simulink model "fangzhen20200803"  (Simulink 9.0)
settings: Solver=ode4  StartTime=0.0  StopTime=500  FixedStep=0.05  RelTol=1e-3
InitFcn:
  | data
values from neighbouring files (symbols this model uses):
  A = [1    0     0 ... (first row only)    [cx.m]    (also in data.m = [Wex^2-W^2   Wex*Wey    Wex*Wez; data1.m = [Wex^2-W^2   Wex*Wey    Wex*Wez)
  a = F/m0    (= 0.2)    [data.m]    (also in data1.m = 0.02)
  a0 = 2*a*k/(4*a+k)    (= 0.08)    [data.m]    (also in data1.m = 0.00363636363636)
  AWcc = [1 1 1]*0.15/3600/3*pi/180    [data.m]    (also in data1.m)
  B = [   0    -2*Wez    2*Wey ... (first row only)    [data.m]    (also in data1.m)
  b = 0.00001*(a+a0)/(2*a*a0)    (= 8.75e-05)    [data.m]    (also in data1.m = 0.01625)
  c20 = -0.113    [data.m]    (also in data1.m)
  c22 = 0.0396    [data.m]    (also in data1.m)
  CWw = [1,1,1,1]*6e-5    [data.m]    (also in data1.m)
  d = 0.01    [data.m]    (also in data1.m = 0.1)
  DWN = [sin(bata)*cos(alpha)  sin(bata)*sin(alpha)  -sin(bata)*cos(alpha)  -sin(bata)*sin(alpha) ... (first row only)    [data.m]    (also in data1.m)
  f = f+2*pi    [E2C.m]    (also in data.m = -0.02; data1.m = 0.02)
  Gl = [-cos(xit0)*sin(fai0)   sin(xit0)*sin(fai0)    cos(fai0) ... (first row only)    [data.m]    (also in data1.m)
  HBd0 = IBd*We0    [data.m]    (also in data1.m)
  Hwmax = JW.*Wwmax    [data.m]    (also in data1.m)
  HWw0 = [0.01 0.01 0.01 0.01]    [data.m]    (also in data1.m)
  InvIBd = inv(IBd)    [data.m]    (also in data1.m)
  invJW = 1 ./JW    [data.m]    (also in data1.m)
  Isp = 300*9.8    (= 2940)    [data.m]    (also in data1.m)
  IW = [1,1,1,1]*1.e-6    [data.m]    (also in data1.m)
  JW = [1,1,1,1]*0.0017362    [data.m]    (also in data1.m)
  Kd = [19.2895;16.6643;22.1166]    [data.m]    (also in data1.m)
  Ki = [0.0503;0.0503;0.0503]    [data.m]    (also in data1.m)
  Kp = [7.0313;6.0484;8.0898]    [data.m]    (also in data1.m)
  m0 = 200    [data.m]    (also in data1.m)
  Mu = 4.794e3    (= 4794)    [data.m]    (also in data1.m)
  MWN = DWN'*inv(DWN*DWN')    [data.m]    (also in data1.m)
  Noise_gc = [1 -1 1]*6/3600*pi/180    [data.m]    (also in data1.m)
  Noise_gn = ([1 1 1]*0.0025/3.*pi/180).^2    [data.m]    (also in data1.m)
  Noise_rwn = ([1 1 1].*1e-10).^2    [data.m]    (also in data1.m)
  Qb0 = [QQQ(4);QQQ(1:3)]    [data.m]    (also in data1.m)
  r0 = [100;-200;1000]    [data.m]    (also in data1.m = [200;300;1000])
  R0 = Tl*[0;0;R0l]    [data.m]    (also in data1.m)
  re = 1750    [data.m]    (also in data1.m)
  rg0 = [3;-104;950]    [data.m]    (also in data1.m = [203;292;998])
  Rtb = [0;0;0]    [data.m]    (also in data1.m = [-30;50;0])
  T = 200    [data.m]    (also in data1.m = 1200)
  TA = [0 0 0]'    [data.m]    (also in data1.m)
  TB = [500 0 0]'    [data.m]    (also in data1.m)
  TC = [500 500 0]'    [data.m]    (also in data1.m)
  Tcmax = [1,1,1,1].*0.02    [data.m]    (also in data1.m)
  TWf0 = [1,1,1,1]*3e-4    [data.m]    (also in data1.m)
  v0 = [-0.1;0.1;-0.3]    [data.m]    (also in data1.m = [0.1;0.1;-1.0])
  vg0 = [0;-0.1;-0.4]    [data.m]    (also in data1.m = [0;-0.1;-0.7])
  Wcc = [1 1 1]*0.2    [data.m]    (also in data1.m)
  We = Tl*Gl'*[0;0;W]    [data.m]    (also in data1.m)
  Wgmax = 10*[1,1,1]'*pi/180    [data.m]    (also in data1.m)
undefined symbols (not defined in the file or in its folder): DiscIntNeverNeededParam, HB0, magnitude
libraries: sharedtransform x4, aerolibobsolete x4, sharedutil x1
(part 1 of 2)
settings Model: SuppressorTable=22 serialization::archive 11 0 6 0 0 0 0 0  Creator=Administrator  LastModifiedBy=chenshiming
settings DataIOCC: LimitDataPoints=on  SignalLoggingSaveFormat=ModelDataLogs  SignalLoggingName=sigsOut
settings OptimizationCC: BlockReduction=off  DefaultParameterBehavior=Inlined  BufferReuse=off  ExpressionDepthLimit=2147483647
settings DebuggingCC: SaveWithParameterizedLinksMsg=none  SignalResolutionControl=TryResolveAllWithWarning  MultiTaskDSMMsg=warning  MultiTaskCondExecSysMsg=none  StateNameClashWarn=warning  StrictBusMsg=None
settings HardwareCC: TargetBitPerLong=64  TargetBitPerPointer=64  TargetBitPerSizeT=64  TargetBitPerPtrDiffT=64  TargetLongLongMode=on  TargetIntDivRoundTo=Zero  TargetEndianess=LittleEndian  TargetWordSize=64  TargetHWDeviceType=MATLAB Host  ProdEqTarget=off
settings GRTTargetCC: GeneratePreprocessorConditionals=Disable all  CombineOutputUpdateFcns=off  GRTInterface=on

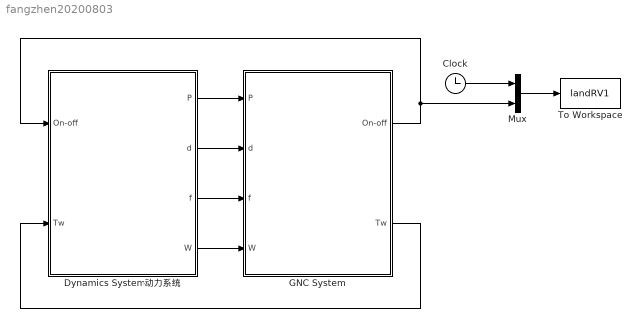
== system fangzhen20200803 ==
  Clock : Clock
  Dynamics System动力系统 : Subsystem
  GNC System : Subsystem
  Mux : Mux  Inputs=2
  To Workspace : ToWorkspace  VariableName=landRV1  SampleTime=-1
  wires:
  Dynamics System动力系统/1(P) -> GNC System/1(P)
  Dynamics System动力系统/2(d) -> GNC System/2(d)
  Dynamics System动力系统/3(f) -> GNC System/3(f)
  Dynamics System动力系统/4(W) -> GNC System/4(W)
  GNC System/1(On-off) -> Dynamics System动力系统/1(On-off), Mux/2
  GNC System/2(Tw) -> Dynamics System动力系统/2(Tw)
  Clock/1 -> Mux/1
  Mux/1 -> To Workspace/1

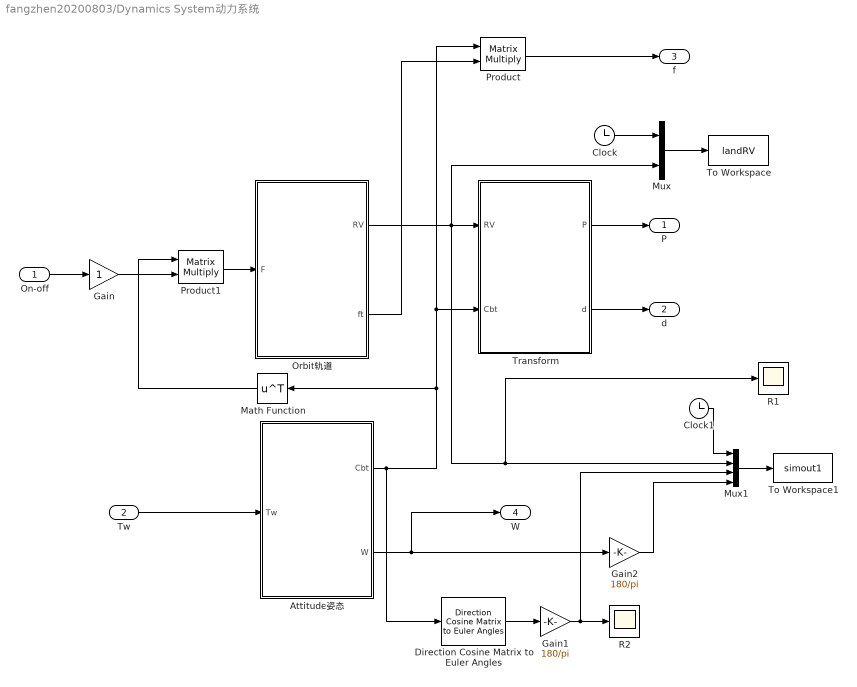
== system fangzhen20200803/Dynamics System动力系统 ==
  On-off : Inport
  Tw : Inport  Port=2
  Attitude姿态 : Subsystem
  Clock : Clock
  Clock1 : Clock
  Direction Cosine Matrix to Euler Angles : aerolibobsolete/Direction Cosine Matrix to Euler Angles
      settings: SourceProductName=Aerospace Blockset  SourceProductBaseCode=AE
  Gain : Gain  SaturateOnIntegerOverflow=on  OutDataTypeStr=Inherit: Same as input  ParamDataTypeStr=Inherit: Same as input
  Gain1 : Gain  Gain=180/pi  SaturateOnIntegerOverflow=on  OutDataTypeStr=Inherit: Same as input  ParamDataTypeStr=Inherit: Same as input
  Gain2 : Gain  Gain=180/pi  SaturateOnIntegerOverflow=on  OutDataTypeStr=Inherit: Same as input  ParamDataTypeStr=Inherit: Same as input
  Math Function : Math  Operator=transpose  SaturateOnIntegerOverflow=on
  Mux : Mux  Inputs=2
  Mux1 : Mux
  Orbit轨道 : Subsystem
  Product : Product  Multiplication=Matrix(*)  SaturateOnIntegerOverflow=on  OutDataTypeStr=Inherit: Same as first input
  Product1 : Product  Multiplication=Matrix(*)  SaturateOnIntegerOverflow=on  OutDataTypeStr=Inherit: Same as first input
  R1 : Scope
  R2 : Scope
  To Workspace : ToWorkspace  VariableName=landRV  SampleTime=-1
  To Workspace1 : ToWorkspace  VariableName=simout1  SampleTime=-1
  Transform : Subsystem
  P : Outport
  d : Outport  Port=2
  f : Outport  Port=3
  W : Outport  Port=4
  wires:
  Tw/1 -> Attitude姿态/1(Tw)
  Attitude姿态/1(Cbt) -> Product/1, Transform/2(Cbt), Math Function/1, Direction Cosine Matrix to Euler Angles/1
  Orbit轨道/2(ft) -> Product/2
  Product/1 -> f/1
  Attitude姿态/2(W) -> W/1, Gain2/1
  Orbit轨道/1(RV) -> R1/1, Mux1/2, Mux/2, Transform/1(RV)
  Transform/2(d) -> d/1
  Transform/1(P) -> P/1
  On-off/1 -> Gain/1
  Product1/1 -> Orbit轨道/1(F)
  Gain/1 -> Product1/2
  Math Function/1 -> Product1/1
  Direction Cosine Matrix to Euler Angles/1 -> Gain1/1
  Gain1/1 -> R2/1, Mux1/3
  Clock/1 -> Mux/1
  Mux/1 -> To Workspace/1
  Clock1/1 -> Mux1/1
  Mux1/1 -> To Workspace1/1
  Gain2/1 -> Mux1/4

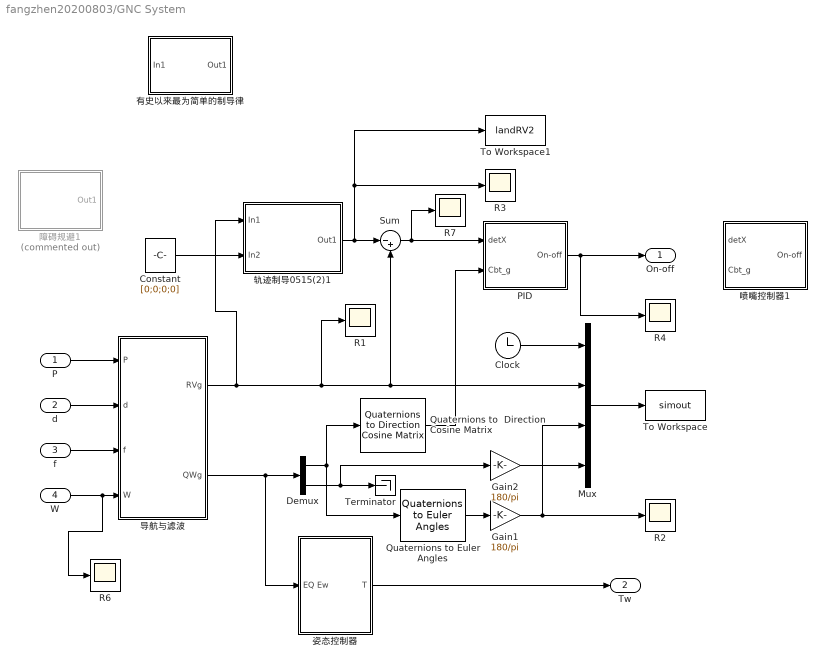
== system fangzhen20200803/GNC System ==
  P : Inport
  d : Inport  Port=2
  f : Inport  Port=3
  W : Inport  Port=4
  Clock : Clock
  Constant : Constant  Value=[0;0;0;0]  VectorParams1D=off
  Demux : Demux  Outputs=[4 3]
  Gain1 : Gain  Gain=180/pi  SaturateOnIntegerOverflow=on  OutDataTypeStr=Inherit: Same as input  ParamDataTypeStr=Inherit: Same as input
  Gain2 : Gain  Gain=180/pi  SaturateOnIntegerOverflow=on  OutDataTypeStr=Inherit: Same as input  ParamDataTypeStr=Inherit: Same as input
  Mux : Mux
  "PID " : Subsystem
  Quaternions to  Direction Cosine Matrix : sharedtransform/Quaternions to  Direction Cosine Matrix
      settings: SourceProductName=Aerospace Blockset  SourceProductBaseCode=AE
  Quaternions to Euler Angles : aerolibobsolete/Quaternions to Euler Angles
      settings: SourceProductName=Aerospace Blockset  SourceProductBaseCode=AE
  R{1..4,6..7} (6 alike) : Scope
  Sum : Sum  Inputs=|-+  SaturateOnIntegerOverflow=on
  Terminator : Terminator
  To Workspace : ToWorkspace  VariableName=simout  SampleTime=-1
  To Workspace1 : ToWorkspace  VariableName=landRV2  SampleTime=-1
  喷嘴控制器1 : Subsystem
  姿态控制器 : Subsystem
      mask help:
      | 输入:
      | 偏差四元数与偏差角速度(本体系下)
      | 输出:
      | 控制电压
      mask Display: disp('姿态控制器')
  导航与滤波 : Subsystem
  "有史以来最为简单的制导律 " : Subsystem
  轨迹制导0515(2)1 : Subsystem
      mask Display: disp('轨迹制导')
  障碍规避1 : Subsystem  Commented=on
      mask Display: disp('障碍规避')
  On-off : Outport
  Tw : Outport  Port=2
  wires:
  P/1 -> 导航与滤波/1(P)
  d/1 -> 导航与滤波/2(d)
  f/1 -> 导航与滤波/3(f)
  W/1 -> R6/1, 导航与滤波/4(W)
  导航与滤波/2(QWg) -> Demux/1, 姿态控制器/1(EQ Ew)
  姿态控制器/1(T) -> Tw/1
  导航与滤波/1(RVg) -> 轨迹制导0515(2)1/1(In1), R1/1, Sum/2, Mux/2
  Demux/2 -> Terminator/1, Gain2/1
  Demux/1 -> Quaternions to  Direction Cosine Matrix/1, Quaternions to Euler Angles/1
  Quaternions to  Direction Cosine Matrix/1 -> "PID "/2(Cbt_g)
  "PID "/1(On-off) -> On-off/1, R4/1
  Quaternions to Euler Angles/1 -> Gain1/1
  Gain1/1 -> R2/1, Mux/3
  Clock/1 -> Mux/1
  Mux/1 -> To Workspace/1
  Gain2/1 -> Mux/4
  Sum/1 -> R7/1, "PID "/1(detX)
  轨迹制导0515(2)1/1(Out1) -> To Workspace1/1, R3/1, Sum/1
  Constant/1 -> 轨迹制导0515(2)1/2(In2)

== system fangzhen20200803/Dynamics System动力系统/Attitude姿态 ==
  Tw : Inport
  Constant : Constant  Value=We
  Product : Product  Multiplication=Matrix(*)  SaturateOnIntegerOverflow=on  OutDataTypeStr=Inherit: Same as first input
  Quaternions to  Direction Cosine Matrix : sharedtransform/Quaternions to  Direction Cosine Matrix
      settings: SourceProductName=Aerospace Blockset  SourceProductBaseCode=AE
  Sum1 : Sum  Inputs=+-  SaturateOnIntegerOverflow=on
  反作用飞轮 : Subsystem
      mask help:
      | 输入:
      | 1、控制信号(力矩形式)
      | 2、星体绝对角速度(本体系下)
      | 输出:
      | 反作用力矩(本体系下)
      mask Display: disp('反作用飞轮')
  姿态动力学模型 : Subsystem
      mask help:
      | 输入:
      | 作用力矩(本体系下)
      | 输出:
      | 绝对角速度(本体系下)
      mask Display: disp('姿态动力学模型')
  星体运动学 : Subsystem  mask(Kinemitics Mask){}
      mask help:
      | 输入:
      | 本体系相对特征点系的角速度(本体系下)
      | 输出:
      | 本体系相对特征点系的姿态四元数
      mask Display: disp('姿态运动学\n(四元数)')
  Cbt : Outport
  W : Outport  Port=2
  wires:
  Tw/1 -> 反作用飞轮/1(Uwheel)
  Quaternions to  Direction Cosine Matrix/1 -> Product/1, Cbt/1
  Constant/1 -> Product/2
  Product/1 -> Sum1/2
  姿态动力学模型/1(Wb) -> Sum1/1, 反作用飞轮/2(Wb), W/1
  Sum1/1 -> 星体运动学/1(In2)
  星体运动学/1(Out2) -> Quaternions to  Direction Cosine Matrix/1
  反作用飞轮/1(TW) -> 姿态动力学模型/1(Torque)

== system fangzhen20200803/Dynamics System动力系统/Orbit轨道 ==
  F : Inport
  轨道动力学模型 : Subsystem
      mask help:
      | 输入:
      | 喷嘴产生的推力(特征点坐标系)
      | 输出:
      | 1、探测器的位置与速度(特征点坐标系)
      | 2、比力(特征点坐标系)
      mask Display: disp('轨道动力学模型')
  RV : Outport
  ft : Outport  Port=2
  wires:
  F/1 -> 轨道动力学模型/1(F)
  轨道动力学模型/1(X) -> RV/1
  轨道动力学模型/2(bl) -> ft/1

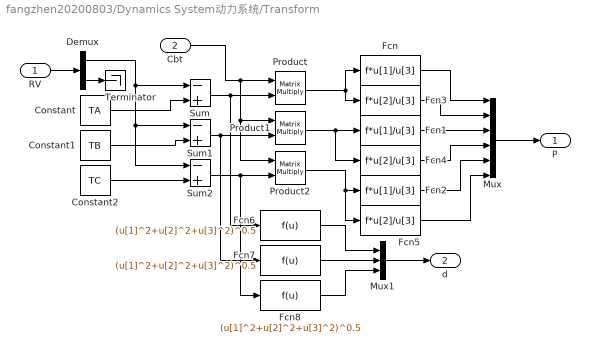
== system fangzhen20200803/Dynamics System动力系统/Transform ==
  RV : Inport
  Cbt : Inport  Port=2
  Constant : Constant  Value=TA
  Constant1 : Constant  Value=TB
  Constant2 : Constant  Value=TC
  Demux : Demux  Outputs=[3 3]
  Fcn : Fcn  Expr=f*u[1]/u[3]
  Fcn1 : Fcn  Expr=f*u[1]/u[3]
  Fcn2 : Fcn  Expr=f*u[1]/u[3]
  Fcn3 : Fcn  Expr=f*u[2]/u[3]
  Fcn4 : Fcn  Expr=f*u[2]/u[3]
  Fcn5 : Fcn  Expr=f*u[2]/u[3]
  Fcn6 : Fcn  Expr=(u[1]^2+u[2]^2+u[3]^2)^0.5
  Fcn7 : Fcn  Expr=(u[1]^2+u[2]^2+u[3]^2)^0.5
  Fcn8 : Fcn  Expr=(u[1]^2+u[2]^2+u[3]^2)^0.5
  Mux : Mux  Inputs=6
  Mux1 : Mux  Inputs=3
  Product : Product  Multiplication=Matrix(*)  SaturateOnIntegerOverflow=on  OutDataTypeStr=Inherit: Same as first input
  Product1 : Product  Multiplication=Matrix(*)  SaturateOnIntegerOverflow=on  OutDataTypeStr=Inherit: Same as first input
  Product2 : Product  Multiplication=Matrix(*)  SaturateOnIntegerOverflow=on  OutDataTypeStr=Inherit: Same as first input
  Sum : Sum  Inputs=-+  SaturateOnIntegerOverflow=on
  Sum1 : Sum  Inputs=-+  SaturateOnIntegerOverflow=on
  Sum2 : Sum  Inputs=-+  SaturateOnIntegerOverflow=on
  Terminator : Terminator
  P : Outport
  d : Outport  Port=2
  wires:
  RV/1 -> Demux/1
  Demux/2 -> Terminator/1
  Demux/1 -> Sum/1, Sum2/1, Sum1/1
  Constant/1 -> Sum/2
  Constant1/1 -> Sum1/2
  Constant2/1 -> Sum2/2
  Cbt/1 -> Product/1, Product2/1, Product1/1
  Sum/1 -> Product/2, Fcn6/1
  Sum1/1 -> Product1/2, Fcn7/1
  Sum2/1 -> Product2/2, Fcn8/1
  Product/1 -> Fcn/1, Fcn3/1
  Product1/1 -> Fcn1/1, Fcn4/1
  Product2/1 -> Fcn2/1, Fcn5/1
  Mux/1 -> P/1
  Fcn7/1 -> Mux1/2
  Fcn8/1 -> Mux1/3
  Fcn6/1 -> Mux1/1
  Mux1/1 -> d/1
  Fcn/1 -> Mux/1
  Fcn3/1 -> Mux/2
  Fcn1/1 -> Mux/3
  Fcn4/1 -> Mux/4
  Fcn2/1 -> Mux/5
  Fcn5/1 -> Mux/6

== system fangzhen20200803/GNC System/PID  ==
  detX : Inport
  Cbt_g : Inport  Port=2
  Delay : Delay  DelayLength=1  InitialCondition=0  SampleTime=0.05
  Demux : Demux  Outputs=[3 3]
  KD : Gain  Gain=0.01
  KD1 : Gain  Gain=-1
  KP : Gain  Gain=0.0002
  Ki : Gain  Gain=0.03  SaturateOnIntegerOverflow=on  OutDataTypeStr=Inherit: Same as input  ParamDataTypeStr=Inherit: Same as input
  Product : Product  Multiplication=Matrix(*)  SaturateOnIntegerOverflow=on  OutDataTypeStr=Inherit: Same as first input
  Product2 : Product  Multiplication=Matrix(*)  SaturateOnIntegerOverflow=on  OutDataTypeStr=Inherit: Same as first input
  Saturation : Saturate  UpperLimit=[0.01,;0.01; 0.01]  LowerLimit=[-0.01; -0.01; -0.01]
  Scope : Scope
  Scope1 : Scope
  Sum1 : Sum  Inputs=|+|+|  SaturateOnIntegerOverflow=on  InputSameDT=on  OutDataTypeStr=Inherit: Same as first input
  Sum2 : Sum  Inputs=|+|+|+|  SaturateOnIntegerOverflow=on  InputSameDT=on  OutDataTypeStr=Inherit: Same as first input
  Zero-Order Hold : ZeroOrderHold  SampleTime=0.05
  On-off : Outport
  wires:
  detX/1 -> Scope/1, Zero-Order Hold/1
  Demux/1 -> Product/2
  Cbt_g/1 -> Product/1, Product2/1
  Demux/2 -> Product2/2
  Sum2/1 -> On-off/1
  Zero-Order Hold/1 -> KD1/1, Scope1/1
  Product2/1 -> KD/1
  Product/1 -> Sum1/2, KP/1, Delay/1
  Sum1/1 -> Ki/1
  Ki/1 -> Saturation/1
  KD/1 -> Sum2/3
  KP/1 -> Sum2/2
  Delay/1 -> Sum1/1
  Saturation/1 -> Sum2/1
  KD1/1 -> Demux/1

== system fangzhen20200803/GNC System/喷嘴控制器1 ==
  detX : Inport
  Cbt_g : Inport  Port=2
  Clock : Clock
  Constant : Constant  Value=T
  Constant3 : Constant  Value=[(2*a*a0/(a+a0)*b)^0.5;(2*a*a0/(a+a0)*b)^0.5;(2*a*a0/(a+a0)*b)^0.5]
  Demux : Demux  Outputs=[3 3]
  Gain : Gain  Gain=-1  SaturateOnIntegerOverflow=on  OutDataTypeStr=Inherit: Same as input  ParamDataTypeStr=Inherit: Same as input
  Product : Product  Multiplication=Matrix(*)  SaturateOnIntegerOverflow=on  OutDataTypeStr=Inherit: Same as first input
  Product2 : Product  Multiplication=Matrix(*)  SaturateOnIntegerOverflow=on  OutDataTypeStr=Inherit: Same as first input
  Product3 : Product  SaturateOnIntegerOverflow=on  OutDataTypeStr=Inherit: Same as first input
  Relational Operator : RelationalOperator  Operator=<=  RndMeth=Nearest
  Relational Operator3 : RelationalOperator  RndMeth=Nearest
  Relational Operator4 : RelationalOperator  RndMeth=Nearest
  Scope : Scope
  Scope1 : Scope
  Sum1 : Sum  SaturateOnIntegerOverflow=on
  Zero-Order Hold : ZeroOrderHold  SampleTime=0.05
  detR+ : Subsystem
  detR- : Subsystem
  On-off : Outport
  wires:
  Gain/1 -> Relational Operator3/2
  Relational Operator3/1 -> detR-/3(change)
  Relational Operator4/1 -> detR+/3(change)
  detR-/1(-T) -> Sum1/1
  detR+/1(+T) -> Sum1/2
  Constant3/1 -> Gain/1, Relational Operator4/2
  Sum1/1 -> Product3/1
  detX/1 -> Scope/1, Zero-Order Hold/1
  Demux/1 -> Product/2
  Cbt_g/1 -> Product/1, Product2/1
  Product/1 -> detR-/1(detR), detR+/1(detR)
  Demux/2 -> Product2/2
  Product2/1 -> Relational Operator4/1, Relational Operator3/1, detR-/2(detV), detR+/2(detV)
  Clock/1 -> Relational Operator/1
  Constant/1 -> Relational Operator/2
  Relational Operator/1 -> Product3/2
  Product3/1 -> On-off/1
  Zero-Order Hold/1 -> Scope1/1, Demux/1

== system fangzhen20200803/GNC System/姿态控制器 ==
  note: 期望力矩
  note: 飞轮分配力矩
  note: 四元数矢量
  EQ Ew : Inport
  Constant1 : Constant  Value=[0 0 0]
  Demux : Demux  Outputs=[1 3]
  Demux1 : Demux  Outputs=[4 3]
  Discrete-Time Integrator : DiscreteIntegrator  IntegratorMethod=Integration: Backward Euler  InitialConditionSource=external  SampleTime=0.2  ICPrevOutput=DiscIntNeverNeededParam  ICPrevScaledInput=DiscIntNeverNeededParam
  Gain : Gain  Gain=[-1 -1 -1]  SaturateOnIntegerOverflow=on  OutDataTypeStr=Inherit: Same as input  ParamDataTypeStr=Inherit: Same as input
  Kd : Gain  Gain=Kd  SaturateOnIntegerOverflow=on  OutDataTypeStr=Inherit: Same as input  ParamDataTypeStr=Inherit: Same as input
  Ki : Gain  Gain=Ki  SaturateOnIntegerOverflow=on  OutDataTypeStr=Inherit: Same as input  ParamDataTypeStr=Inherit: Same as input
  Kp : Gain  Gain=Kp  SaturateOnIntegerOverflow=on  OutDataTypeStr=Inherit: Same as input  ParamDataTypeStr=Inherit: Same as input
  MWN : Gain  Gain=MWN  Multiplication=Matrix(K*u)  SaturateOnIntegerOverflow=on  OutDataTypeStr=Inherit: Same as input  ParamDataTypeStr=Inherit: Same as input
  Product5 : Product  OutDataTypeStr=double  SaturateOnIntegerOverflow=on  InputSameDT=on
  R1 : Scope
  Saturation : Saturate  UpperLimit=[0.01, 0.01, 0.01]  LowerLimit=[-0.01, -0.01, -0.01]
  Sign : Signum
  Sum : Sum  Inputs=+-  SaturateOnIntegerOverflow=on  InputSameDT=on  OutDataTypeStr=Inherit: Same as first input
  Sum1 : Sum  Inputs=+-  SaturateOnIntegerOverflow=on  InputSameDT=on  OutDataTypeStr=Inherit: Same as first input
  Sum2 : Sum  Inputs=|+|+|+|  SaturateOnIntegerOverflow=on  InputSameDT=on  OutDataTypeStr=Inherit: Same as first input
  Terminator : Terminator
  T : Outport
  wires:
  Sum/1 -> Discrete-Time Integrator/1, Kp/1
  Sum1/1 -> Kd/1
  Discrete-Time Integrator/1 -> Ki/1
  Ki/1 -> Saturation/1
  Kp/1 -> Sum2/2
  Kd/1 -> Sum2/3
  Demux/2 -> Product5/2
  Demux/1 -> Sign/1
  Product5/1 -> Sum/2
  Constant1/1 -> Discrete-Time Integrator/2, Sum1/1, Sum/1
  Sum2/1 -> R1/1, Gain/1
  Demux1/2 -> Sum1/2
  Demux1/1 -> Demux/1
  EQ Ew/1 -> Demux1/1
  Sign/1 -> Product5/1
  Saturation/1 -> Terminator/1, Sum2/1
  MWN/1 -> T/1
  Gain/1 -> MWN/1

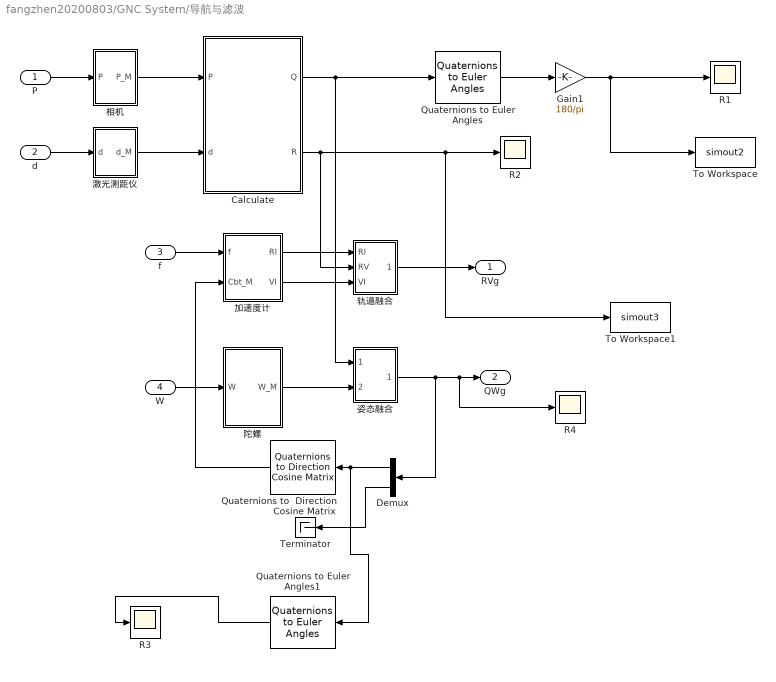
== system fangzhen20200803/GNC System/导航与滤波 ==
  P : Inport
  d : Inport  Port=2
  f : Inport  Port=3
  W : Inport  Port=4
  Calculate : Subsystem
  Demux : Demux  Outputs=[4 3]
  Gain1 : Gain  Gain=180/pi  SaturateOnIntegerOverflow=on  OutDataTypeStr=Inherit: Same as input  ParamDataTypeStr=Inherit: Same as input
  Quaternions to  Direction Cosine Matrix : sharedtransform/Quaternions to  Direction Cosine Matrix
      settings: SourceProductName=Aerospace Blockset  SourceProductBaseCode=AE
  Quaternions to Euler Angles : aerolibobsolete/Quaternions to Euler Angles
      settings: SourceProductName=Aerospace Blockset  SourceProductBaseCode=AE
  Quaternions to Euler Angles1 : aerolibobsolete/Quaternions to Euler Angles
      settings: SourceProductName=Aerospace Blockset  SourceProductBaseCode=AE
  R{1..4} (4 alike) : Scope
  Terminator : Terminator
  To Workspace : ToWorkspace  VariableName=simout2  SampleTime=-1
  To Workspace1 : ToWorkspace  VariableName=simout3  SampleTime=-1
  加速度计 : Subsystem
  姿态融合 : Subsystem
  激光测距仪 : Subsystem
  相机 : Subsystem
  轨道融合 : Subsystem
  陀螺 : Subsystem
  RVg : Outport
  QWg : Outport  Port=2
  wires:
  f/1 -> 加速度计/1(f)
  W/1 -> 陀螺/1(W)
  加速度计/1(RI) -> 轨道融合/1(RI)
  加速度计/2(VI) -> 轨道融合/3(VI)
  Calculate/2(R) -> 轨道融合/2(RV), To Workspace1/1, R2/1
  Calculate/1(Q) -> 姿态融合/1(Q-M), Quaternions to Euler Angles/1
  陀螺/1(W_M) -> 姿态融合/2(w-M)
  轨道融合/1(RVg) -> RVg/1
  姿态融合/1(QWg) -> R4/1, QWg/1, Demux/1
  Demux/1 -> Quaternions to Euler Angles1/1, Quaternions to  Direction Cosine Matrix/1
  Quaternions to  Direction Cosine Matrix/1 -> 加速度计/2(Cbt_M)
  Demux/2 -> Terminator/1
  Quaternions to Euler Angles/1 -> Gain1/1
  Gain1/1 -> R1/1, To Workspace/1
  d/1 -> 激光测距仪/1(d)
  P/1 -> 相机/1(P)
  相机/1(P_M) -> Calculate/1(P)
  激光测距仪/1(d_M) -> Calculate/2(d)
  Quaternions to Euler Angles1/1 -> R3/1

== system fangzhen20200803/GNC System/有史以来最为简单的制导律  ==
  In1 : Inport
  Clock1 : Clock
  Clock2 : Clock
  Constant1 : Constant  Value=0.0000000001
  Divide : Product  Inputs=*/*
  Relational Operator1 : RelationalOperator  Operator=<=  RndMeth=Nearest
  Scope : Scope
  Subsystem2 : Subsystem
  Subtract : Sum  Inputs=+-
  T : Constant  Value=T
  Out1 : Outport
  wires:
  Relational Operator1/1 -> Subsystem2/Enable
  Clock1/1 -> Relational Operator1/1
  Constant1/1 -> Relational Operator1/2
  In1/1 -> Subsystem2/1(In1)
  Subsystem2/1(Out1) -> Subtract/1, Divide/1
  T/1 -> Divide/2
  Clock2/1 -> Divide/3
  Divide/1 -> Subtract/2
  Subtract/1 -> Scope/1, Out1/1

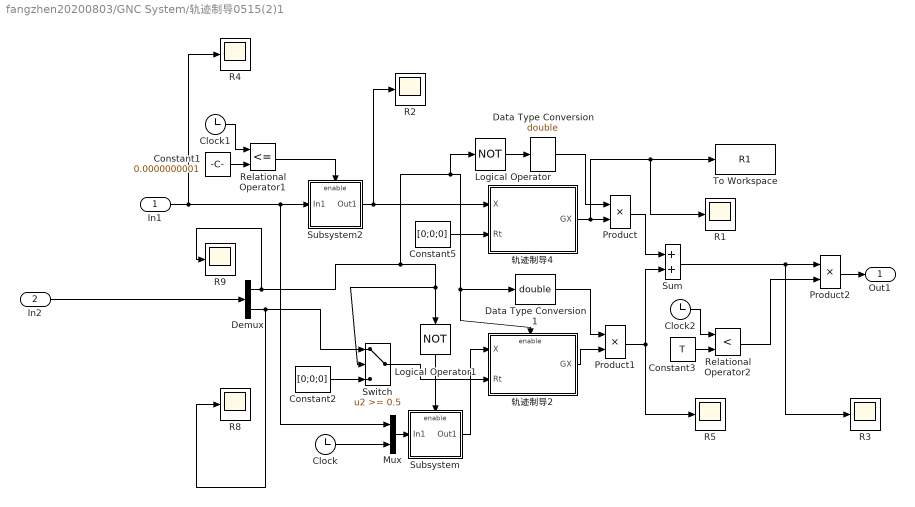
== system fangzhen20200803/GNC System/轨迹制导0515(2)1 ==
  In1 : Inport
  In2 : Inport  Port=2
  Clock : Clock
  Clock1 : Clock
  Clock2 : Clock
  Constant1 : Constant  Value=0.0000000001
  Constant2 : Constant  Value=[0;0;0]
  Constant3 : Constant  Value=T
  Constant5 : Constant  Value=[0;0;0]
  Data Type Conversion : DataTypeConversion  OutDataTypeStr=double  SaturateOnIntegerOverflow=on  RndMeth=Zero
  Data Type Conversion1 : DataTypeConversion  OutDataTypeStr=double  SaturateOnIntegerOverflow=on  RndMeth=Zero
  Demux : Demux  Outputs=[1 3]
  Logical Operator : Logic  Operator=NOT  AllPortsSameDT=off
  Logical Operator1 : Logic  Operator=NOT  AllPortsSameDT=off
  Mux : Mux  Inputs=[6 1]
  Product : Product  SaturateOnIntegerOverflow=on  OutDataTypeStr=Inherit: Same as first input
  Product1 : Product  SaturateOnIntegerOverflow=on  OutDataTypeStr=Inherit: Same as first input
  Product2 : Product  SaturateOnIntegerOverflow=on  OutDataTypeStr=Inherit: Same as first input
  R{1..5,8..9} (7 alike) : Scope
  Relational Operator1 : RelationalOperator  Operator=<=  RndMeth=Nearest
  Relational Operator2 : RelationalOperator  Operator=<  RndMeth=Nearest
  Subsystem : Subsystem
  Subsystem2 : Subsystem
  Sum : Sum  SaturateOnIntegerOverflow=on
  Switch : Switch  Threshold=0.5  SaturateOnIntegerOverflow=on
  To Workspace : ToWorkspace  VariableName=R1  SampleTime=-1
  轨迹制导2 : Subsystem
      mask help:
      | 利用导航量进行轨迹规划(秒钟规划一次)(利用位置、速度约束)(只有Z轴方向进行了规划)
      | 输入:
      | 导航量(位置、速度)
      | 输出:
      | 规划的期望轨迹(位置、速度)
      mask Display: disp('轨迹制导')
  轨迹制导4 : Subsystem
      mask help:
      | 利用导航量进行轨迹规划(秒钟规划一次)(利用位置、速度和加速度约束)
      | 输入:
      | 1 、导航量(位置、速度)
      | 2、 期望终端位置
      | 输出为当前规划的期望轨迹(位置、速度)
      mask Display: disp('轨迹制导')
  Out1 : Outport
  wires:
  Relational Operator2/1 -> Product2/2
  Product2/1 -> Out1/1
  Clock2/1 -> Relational Operator2/1
  Constant3/1 -> Relational Operator2/2
  Demux/2 -> Switch/1, R8/1
  Demux/1 -> Data Type Conversion1/1, 轨迹制导2/Enable, Logical Operator/1, Switch/2, Logical Operator1/1, R9/1
  In2/1 -> Demux/1
  Logical Operator1/1 -> Subsystem/Enable
  Constant5/1 -> 轨迹制导4/2(Rt)
  Constant2/1 -> Switch/3
  Switch/1 -> 轨迹制导2/2(Rt)
  Subsystem2/1(Out1) -> 轨迹制导4/1(X), R2/1
  In1/1 -> Mux/1, Subsystem2/1(In1), R4/1
  Relational Operator1/1 -> Subsystem2/Enable
  Clock1/1 -> Relational Operator1/1
  Constant1/1 -> Relational Operator1/2
  Data Type Conversion1/1 -> Product1/1
  Data Type Conversion/1 -> Product/1
  Product1/1 -> Sum/2, R5/1
  轨迹制导2/1(GX) -> Product1/2
  Subsystem/1(Out1) -> 轨迹制导2/1(X)
  Mux/1 -> Subsystem/1(In1)
  Clock/1 -> Mux/2
  轨迹制导4/1(GX) -> To Workspace/1, R1/1, Product/2
  Product/1 -> Sum/1
  Sum/1 -> R3/1, Product2/1
  Logical Operator/1 -> Data Type Conversion/1

== system fangzhen20200803/GNC System/障碍规避1 ==
  Clock2 : Clock  Commented=on
  Constant : Constant  Value=0  VectorParams1D=off
  Constant3 : Constant  Value=Rtb
  Constant4 : Constant  Commented=on  Value=100000
  Mux : Mux  Inputs=[1,3]
  Relational Operator : RelationalOperator  Commented=on  RndMeth=Nearest
  Out1 : Outport
  wires:
  Mux/1 -> Out1/1
  Constant3/1 -> Mux/2
  Constant4/1 -> Relational Operator/2
  Clock2/1 -> Relational Operator/1
  Constant/1 -> Mux/1

== system fangzhen20200803/Dynamics System动力系统/Attitude姿态/反作用飞轮 ==
  Uwheel : Inport
  Wb : Inport  Port=2
  Torque : Subsystem
  wheelmid : Subsystem
  TW : Outport
  wires:
  wheelmid/1(Ww) -> Torque/1(Ew)
  Wb/1 -> Torque/2(Wb)
  Torque/1(TW) -> TW/1
  Uwheel/1 -> wheelmid/1(Uwheel)

== system fangzhen20200803/Dynamics System动力系统/Attitude姿态/姿态动力学模型 ==
  note: Wb
  note: Hb
  Torque : Inport
  3x3 Cross Product : Subsystem  AncestorBlock=aerolibtransform/3x3 Cross Product  mask(CrossProduct){}
      mask help: Calculate the cross product of two 3-by-1 vectors.
      mask Help: web(asbhelp('3x3crossproduct'));
      mask Display: disp('Cross Product \n C = AxB')
  Constant1 : Constant  Value=HBd0
  Integrator1 : Integrator  InitialConditionSource=external  InitialCondition=HB0
  InvIBu : Gain  Gain=InvIBd  Multiplication=Matrix(K*u)  SaturateOnIntegerOverflow=on  OutDataTypeStr=Inherit: Same as input  ParamDataTypeStr=Inherit: Same as input
  Sum1 : Sum  Inputs=-+  SaturateOnIntegerOverflow=on  InputSameDT=on  OutDataTypeStr=Inherit: Same as first input
  Wb : Outport
  wires:
  Sum1/1 -> Integrator1/1
  Torque/1 -> Sum1/2
  3x3 Cross Product/1(C) -> Sum1/1
  Constant1/1 -> Integrator1/2
  InvIBu/1 -> Wb/1, 3x3 Cross Product/1(A)
  Integrator1/1 -> InvIBu/1, 3x3 Cross Product/2(B)

== system fangzhen20200803/Dynamics System动力系统/Attitude姿态/星体运动学 ==
  In2 : Inport
  3x3 Cross Product : sharedutil/3x3 Cross Product
      settings: SourceProductBaseCode=AE
  Constant3 : Constant  Value=Qb0
  Demux : Demux  Outputs=[1,3]
  Dot Product : DotProduct  InputSameDT=on  OutDataTypeStr=Inherit: Inherit via internal rule
  Gain : Gain  Gain=-0.5  SaturateOnIntegerOverflow=on  OutDataTypeStr=Inherit: Same as input  ParamDataTypeStr=Inherit: Same as input
  Gain1 : Gain  Gain=0.5  SaturateOnIntegerOverflow=on  OutDataTypeStr=Inherit: Same as input  ParamDataTypeStr=Inherit: Same as input
  Integrator : Integrator  InitialConditionSource=external  InitialCondition=Qb0
  Mux : Mux  Inputs=[1,3]
  Product : Product  SaturateOnIntegerOverflow=on  InputSameDT=on  OutDataTypeStr=Inherit: Same as first input
  Sum1 : Sum  SaturateOnIntegerOverflow=on  InputSameDT=on  OutDataTypeStr=Inherit: Same as first input
  Out2 : Outport
  wires:
  Demux/2 -> Dot Product/2, 3x3 Cross Product/1
  Demux/1 -> Product/1
  Integrator/1 -> Out2/1, Demux/1
  Mux/1 -> Integrator/1
  Dot Product/1 -> Gain/1
  Sum1/1 -> Gain1/1
  Gain/1 -> Mux/1
  In2/1 -> Product/2, 3x3 Cross Product/2, Dot Product/1
  Product/1 -> Sum1/2
  Gain1/1 -> Mux/2
  3x3 Cross Product/1 -> Sum1/1
  Constant3/1 -> Integrator/2

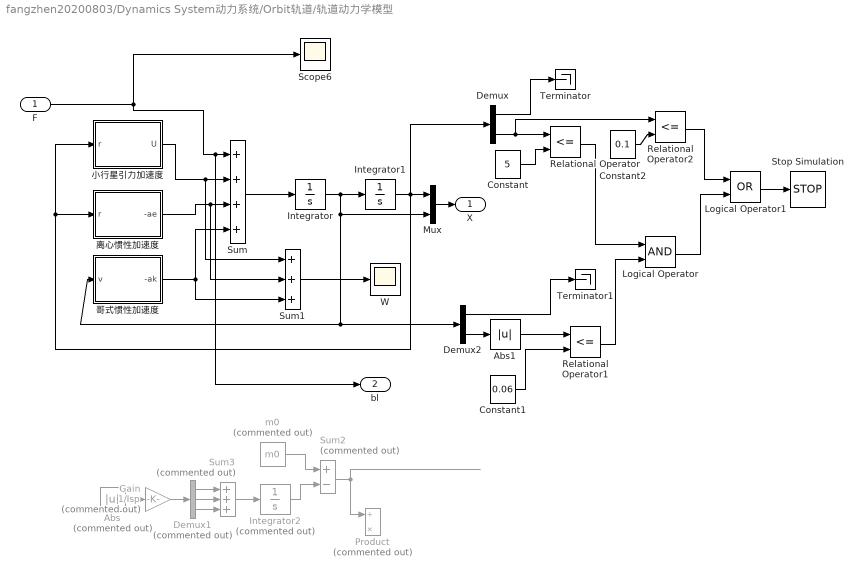
== system fangzhen20200803/Dynamics System动力系统/Orbit轨道/轨道动力学模型 ==
  F : Inport
  Abs : Abs  Commented=on  SaturateOnIntegerOverflow=on
  Abs1 : Abs  SaturateOnIntegerOverflow=on
  Constant : Constant  Value=5
  Constant1 : Constant  Value=0.06
  Constant2 : Constant  Value=0.1
  Demux : Demux  Outputs=[2 1]
  Demux1 : Demux  Commented=on  Outputs=3
  Demux2 : Demux  Outputs=[2 1]
  Gain : Gain  Commented=on  Gain=1/Isp  SaturateOnIntegerOverflow=on  OutDataTypeStr=Inherit: Same as input  ParamDataTypeStr=Inherit: Same as input
  Integrator : Integrator  InitialCondition=v0
  Integrator1 : Integrator  InitialCondition=r0
  Integrator2 : Integrator  Commented=on
  Logical Operator : Logic  AllPortsSameDT=off
  Logical Operator1 : Logic  Operator=OR  AllPortsSameDT=off
  Mux : Mux  Inputs=2
  Product : Product  Commented=on  Inputs=/*  SaturateOnIntegerOverflow=on  OutDataTypeStr=Inherit: Same as first input
  Relational Operator : RelationalOperator  Operator=<=  RndMeth=Nearest
  Relational Operator1 : RelationalOperator  Operator=<=  RndMeth=Nearest
  Relational Operator2 : RelationalOperator  Operator=<=  RndMeth=Nearest
  Scope6 : Scope
  Stop Simulation : Stop
  Sum : Sum  Inputs=++++  SaturateOnIntegerOverflow=on
  Sum1 : Sum  Inputs=+++  SaturateOnIntegerOverflow=on
  Sum2 : Sum  Commented=on  Inputs=+-  SaturateOnIntegerOverflow=on
  Sum3 : Sum  Commented=on  Inputs=+++  SaturateOnIntegerOverflow=on
  Terminator : Terminator
  Terminator1 : Terminator
  W : Scope
  m0 : Constant  Commented=on  Value=m0
  哥式惯性加速度 : Subsystem
  小行星引力加速度 : Subsystem
  离心惯性加速度 : Subsystem
  X : Outport
  bl : Outport  Port=2
  wires:
  小行星引力加速度/1(U) -> Sum/2, Sum1/1
  离心惯性加速度/1(-ae) -> Sum/3, Sum1/2
  哥式惯性加速度/1(-ak) -> Sum/4, Sum1/3
  Sum/1 -> Integrator/1
  Integrator/1 -> Integrator1/1, Mux/2, 哥式惯性加速度/1(v), Demux2/1
  Mux/1 -> X/1
  Integrator1/1 -> Mux/1, Demux/1, 离心惯性加速度/1(r), 小行星引力加速度/1(r)
  Demux/1 -> Terminator/1
  Demux/2 -> Relational Operator/1, Relational Operator2/1
  Constant/1 -> Relational Operator/2
  F/1 -> Sum/1, bl/1, Scope6/1
  Sum1/1 -> W/1
  Demux2/1 -> Terminator1/1
  Demux2/2 -> Abs1/1
  Constant1/1 -> Relational Operator1/2
  Relational Operator1/1 -> Logical Operator/2
  Relational Operator/1 -> Logical Operator/1
  Abs1/1 -> Relational Operator1/1
  Logical Operator/1 -> Logical Operator1/2
  Logical Operator1/1 -> Stop Simulation/1
  Constant2/1 -> Relational Operator2/2
  Relational Operator2/1 -> Logical Operator1/1
  Abs/1 -> Gain/1
  Sum3/1 -> Integrator2/1
  Demux1/1 -> Sum3/1
  Demux1/2 -> Sum3/2
  Sum2/1 -> Product/1
  Integrator2/1 -> Sum2/2
  m0/1 -> Sum2/1
  Demux1/3 -> Sum3/3
  ? -> Abs/1
  ? -> Product/2
  Gain/1 -> Demux1/1

== system fangzhen20200803/GNC System/喷嘴控制器1/detR+ ==
  detR : Inport
  detV : Inport  Port=2
  change : Inport  Port=3
  AND : Logic  AllPortsSameDT=off
  AND1 : Logic  AllPortsSameDT=off
  Gain : Gain  SaturateOnIntegerOverflow=on  OutDataTypeStr=Inherit: Same as input  ParamDataTypeStr=Inherit: Same as input
  NOT : Logic  Operator=NOT  AllPortsSameDT=off
  Relational Operator1 : RelationalOperator  Operator=<  RndMeth=Nearest
  Relational Operator2 : RelationalOperator  Operator=<=  RndMeth=Nearest
  Sum1 : Sum  OutDataTypeStr=double  SaturateOnIntegerOverflow=on
  Switch : Subsystem
  +T : Outport
  wires:
  Relational Operator1/1 -> AND1/1
  Relational Operator2/1 -> AND/1
  Switch/1(Out1) -> Relational Operator2/2
  Switch/2(Out2) -> Relational Operator1/2
  change/1 -> NOT/1, AND/2
  NOT/1 -> AND1/2
  AND/1 -> Sum1/1
  AND1/1 -> Sum1/2
  Sum1/1 -> Gain/1
  detV/1 -> Switch/1(detV)
  detR/1 -> Relational Operator2/1, Relational Operator1/1
  Gain/1 -> +T/1

== system fangzhen20200803/GNC System/喷嘴控制器1/detR- ==
  detR : Inport
  detV : Inport  Port=2
  change : Inport  Port=3
  AND : Logic  AllPortsSameDT=off
  AND1 : Logic  AllPortsSameDT=off
  Gain1 : Gain  Gain=-1  SaturateOnIntegerOverflow=on  OutDataTypeStr=Inherit: Same as input  ParamDataTypeStr=Inherit: Same as input
  NOT : Logic  Operator=NOT  AllPortsSameDT=off
  Relational Operator1 : RelationalOperator  Operator=>  RndMeth=Nearest
  Relational Operator2 : RelationalOperator  RndMeth=Nearest
  Sum1 : Sum  OutDataTypeStr=double  SaturateOnIntegerOverflow=on
  Switch : Subsystem
  -T : Outport
  wires:
  Relational Operator1/1 -> AND1/1
  Relational Operator2/1 -> AND/1
  Switch/1(Out1) -> Relational Operator2/2
  Switch/2(Out2) -> Relational Operator1/2
  detR/1 -> Relational Operator1/1, Relational Operator2/1
  change/1 -> NOT/1, AND/2
  NOT/1 -> AND1/2
  AND/1 -> Sum1/1
  AND1/1 -> Sum1/2
  Sum1/1 -> Gain1/1
  detV/1 -> Switch/1(detV)
  Gain1/1 -> -T/1

== system fangzhen20200803/GNC System/导航与滤波/Calculate ==
  P : Inport
  d : Inport  Port=2
  Demux : Demux  Outputs=[2 2 2]
  Demux1 : Demux  Outputs=[1 1 1]
  Mux : Mux  Inputs=2
  Mux1 : Mux  Inputs=2
  Mux2 : Mux  Inputs=2
  P1 : Subsystem
  P2 : Subsystem
  P3 : Subsystem
  Subsystem3 : Subsystem
  Q : Outport
  R : Outport  Port=2
  wires:
  P1/1(Out1) -> Subsystem3/1(In1)
  P2/1(Out1) -> Subsystem3/2(In2)
  P3/1(Out1) -> Subsystem3/3(In3)
  Subsystem3/2(Q) -> Q/1
  Subsystem3/1(R) -> R/1
  P/1 -> Demux/1
  d/1 -> Demux1/1
  Demux/1 -> Mux/1
  Demux1/1 -> Mux/2
  Demux/2 -> Mux1/1
  Demux1/2 -> Mux1/2
  Demux1/3 -> Mux2/2
  Demux/3 -> Mux2/1
  Mux/1 -> P1/1(In1)
  Mux1/1 -> P2/1(In1)
  Mux2/1 -> P3/1(In1)

== system fangzhen20200803/GNC System/导航与滤波/加速度计 ==
  f : Inport
  Cbt_M : Inport  Port=2
  Integrator : Integrator  InitialCondition=vg0
  Integrator1 : Integrator  InitialCondition=rg0
  Math Function : Math  Operator=transpose  SaturateOnIntegerOverflow=on
  Product1 : Product  Multiplication=Matrix(*)  SaturateOnIntegerOverflow=on  OutDataTypeStr=Inherit: Same as first input
  R2 : Scope
  Random Number : RandomNumber  Commented=on  Mean=[0 0 0]  Variance=[1.2185e-004 1.2185e-004 1.2185e-004]  Seed=[15683 12482 12355]  SampleTime=0
  Sum2 : Sum  Inputs=+++  SaturateOnIntegerOverflow=on
  cp : Constant  Value=[0 0 0]
  RI : Outport
  VI : Outport  Port=2
  wires:
  Product1/1 -> Integrator/1
  Math Function/1 -> Product1/1
  Cbt_M/1 -> Math Function/1
  f/1 -> Sum2/1
  cp/1 -> Sum2/3
  Integrator1/1 -> RI/1, R2/1
  Integrator/1 -> VI/1, Integrator1/1
  Sum2/1 -> Product1/2
  Random Number/1 -> Sum2/2

== system fangzhen20200803/GNC System/导航与滤波/姿态融合 ==
  Q-M : Inport
  w-M : Inport  Port=2
  Mux : Mux  Inputs=[4 3]
  S-Function : S-Function  Commented=on  FunctionName=CIQW_kf_C  SFunctionDeploymentMode=off  EnableBusSupport=off
  QWg : Outport
  wires:
  Mux/1 -> QWg/1
  Q-M/1 -> Mux/1
  w-M/1 -> Mux/2

== system fangzhen20200803/GNC System/导航与滤波/激光测距仪 ==
  d : Inport
  Abs : Abs  SaturateOnIntegerOverflow=on
  Gain : Gain  Gain=11
  Random Number : RandomNumber  Commented=on  Mean=[0 0 0]  Variance=[10 10 10]  Seed=[15683 12482 12355]  SampleTime=0
  Sine Wave : Sin  SampleTime=0
  Sum6 : Sum  SaturateOnIntegerOverflow=on
  d_M : Outport
  wires:
  d/1 -> Sum6/1
  Sum6/1 -> Abs/1
  Abs/1 -> d_M/1
  Sine Wave/1 -> Gain/1
  Random Number/1 -> Sum6/2

== system fangzhen20200803/GNC System/导航与滤波/相机 ==
  P : Inport
  Gain : Gain  Commented=on  Gain=0.0001
  Random Number : RandomNumber  Commented=on  Mean=[0 0 0 0 0 0]  Variance=[1e-8 1e-8 1e-8 1e-8 1e-8 1e-8]  Seed=[15683 12482 12355 15000 12000 12000]  SampleTime=0
  Scope : Scope  Commented=on
  Sine Wave : Sin  Commented=on  SampleTime=0
  Sum6 : Sum  SaturateOnIntegerOverflow=on
  P_M : Outport
  wires:
  Sum6/1 -> P_M/1
  P/1 -> Sum6/1
  Sine Wave/1 -> Gain/1
  Random Number/1 -> Sum6/2
  Gain/1 -> Scope/1

== system fangzhen20200803/GNC System/导航与滤波/轨道融合 ==
  RI : Inport
  RV : Inport  Port=2
  VI : Inport  Port=3
  Demux1 : Demux  Commented=on  Outputs=[3 3]
  Mux : Mux  Inputs=[3 3]
  Mux1 : Mux  Inputs=[3 3]
  S-Function : S-Function  Commented=on  FunctionName=CIRV_kf_C  SFunctionDeploymentMode=off  EnableBusSupport=off
  Scope1 : Scope
  Scope5 : Scope
  Sum1 : Sum  Inputs=+-  SaturateOnIntegerOverflow=on
  Sum4 : Sum  Inputs=+-  SaturateOnIntegerOverflow=on
  RVg : Outport
  wires:
  Mux/1 -> S-Function/1
  S-Function/1 -> Demux1/1, Scope5/1
  RI/1 -> Mux/1, Sum4/1
  RV/1 -> Mux/2
  Demux1/1 -> Sum4/2
  VI/1 -> Sum1/1
  Demux1/2 -> Sum1/2
  Sum4/1 -> Mux1/1
  Sum1/1 -> Mux1/2
  Mux1/1 -> Scope1/1, RVg/1

== system fangzhen20200803/GNC System/导航与滤波/陀螺 ==
  W : Inport
  AWcc : Gain  Gain=AWcc  SaturateOnIntegerOverflow=on  OutDataTypeStr=Inherit: Same as input  ParamDataTypeStr=Inherit: Same as input
  Clock : Clock
  Integrator : Integrator  InitialCondition=[0;0;0]
  Mux : Mux  Inputs=3
  Noigc : Constant  Commented=on  Value=Noise_gc
  Noign : RandomNumber  Commented=on  Mean=[0 0 0]  Variance=Noise_gn  Seed=[1859 2483 4682]  SampleTime=0
  Noign1 : RandomNumber  Commented=on  Mean=[0 0 0]  Variance=Noise_rwn  Seed=[4983 1983 6943]  SampleTime=0
  Sum : Sum  Inputs=|+|+|+|+|+  SaturateOnIntegerOverflow=on  InputSameDT=on  OutDataTypeStr=Inherit: Same as first input
  Trigonometric Function : Trigonometry
  Wcc : Gain  Gain=Wcc  SaturateOnIntegerOverflow=on  OutDataTypeStr=Inherit: Same as input  ParamDataTypeStr=Inherit: Same as input
  Wgmax : Saturate  UpperLimit=Wgmax  LowerLimit=-Wgmax
  W_M : Outport
  wires:
  Clock/1 -> Mux/2, Mux/1, Mux/3
  Mux/1 -> Wcc/1
  Wcc/1 -> Trigonometric Function/1
  Trigonometric Function/1 -> AWcc/1
  W/1 -> Wgmax/1
  Wgmax/1 -> Sum/3
  Noign/1 -> Sum/4
  AWcc/1 -> Sum/2
  Noigc/1 -> Sum/1
  Sum/1 -> W_M/1
  Noign1/1 -> Integrator/1
  Integrator/1 -> Sum/5

== system fangzhen20200803/GNC System/有史以来最为简单的制导律 /Subsystem2 ==
  In1 : Inport
  Enable : EnablePort
  Out1 : Outport
  wires:
  In1/1 -> Out1/1

== system fangzhen20200803/GNC System/轨迹制导0515(2)1/Subsystem ==
  In1 : Inport
  Enable : EnablePort
  Out1 : Outport
  wires:
  In1/1 -> Out1/1

== system fangzhen20200803/GNC System/轨迹制导0515(2)1/Subsystem2 ==
  In1 : Inport
  Enable : EnablePort
  Out1 : Outport
  wires:
  In1/1 -> Out1/1

== system fangzhen20200803/GNC System/轨迹制导0515(2)1/轨迹制导2 ==
  X : Inport
  Rt : Inport  Port=2
  Enable : EnablePort
  Clock : Clock
  Constant1 : Constant  Value=[0 0]  OutDataTypeStr=double
  Constant2 : Constant  Value=T  OutDataTypeStr=double
  Demux : Demux  Outputs=[2 1 2 1]
  Demux1 : Demux  Outputs=[6 1]
  Demux2 : Demux  Outputs=[2 1]
  Mux : Mux  Inputs=[2 1 2 1]
  Sum1 : Sum  Inputs=-+  SaturateOnIntegerOverflow=on
  Sum2 : Sum  Inputs=-+  SaturateOnIntegerOverflow=on
  Sum3 : Sum  SaturateOnIntegerOverflow=on
  Sum4 : Sum  Inputs=+-  SaturateOnIntegerOverflow=on
  Terminator : Terminator
  Terminator1 : Terminator
  r : Subsystem
  v : Subsystem
  GX : Outport
  wires:
  Sum4/1 -> Mux/2
  r/1(r) -> Sum4/1
  Sum3/1 -> v/3(r0), r/3(r0)
  Demux/2 -> Sum3/1
  Demux2/2 -> Sum4/2, Sum3/2
  Demux/4 -> v/4(v0), r/4(v0)
  Sum2/1 -> v/2(t), r/2(t)
  Sum1/1 -> v/1(tgo), r/1(tgo)
  Clock/1 -> Sum2/2
  Demux1/2 -> Sum2/1, Sum1/1
  Demux2/1 -> Mux/1
  Rt/1 -> Demux2/1
  Constant2/1 -> Sum1/2
  v/1(v) -> Mux/4
  Demux/3 -> Terminator1/1
  Demux/1 -> Terminator/1
  Constant1/1 -> Mux/3
  Mux/1 -> GX/1
  Demux1/1 -> Demux/1
  X/1 -> Demux1/1

== system fangzhen20200803/GNC System/轨迹制导0515(2)1/轨迹制导4 ==
  note: [0 0 0]
  note: 位置速度
  X : Inport
  Rt : Inport  Port=2
  C0 : Subsystem
  C1 : Subsystem
  C2 : Subsystem
  Clock : Clock
  Demux : Demux  Outputs=[3 3]
  Mux : Mux  Inputs=2
  T : Constant  Value=T
  r : Subsystem
  v : Subsystem
  GX : Outport
  wires:
  X/1 -> Demux/1
  Demux/1 -> C0/1(r), C1/1(r), C2/1(r), r/5(r0)
  Demux/2 -> C0/2(v), C1/2(v), C2/2(v), v/5(v0), r/6(v0)
  C0/1(C0) -> r/1(C0), v/1(C0)
  C1/1(C1) -> r/2(C1), v/2(C1)
  C2/1(C2) -> r/3(C2), v/3(C2)
  Clock/1 -> r/4(t), v/4(t)
  Mux/1 -> GX/1
  r/1(r) -> Mux/1
  v/1(v) -> Mux/2
  Rt/1 -> C0/4(rt), C1/4(rt), C2/4(rt)
  T/1 -> C1/3(tgo), C0/3(tgo), C2/3(tgo)

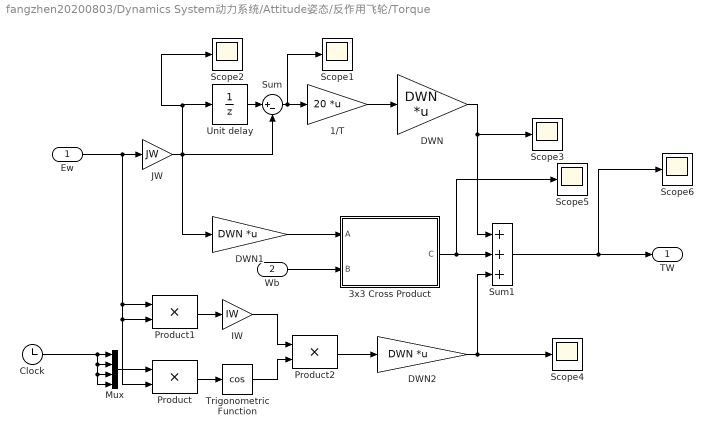
== system fangzhen20200803/Dynamics System动力系统/Attitude姿态/反作用飞轮/Torque ==
  Ew : Inport
  Wb : Inport  Port=2
  1/T : Gain  Gain=20  Multiplication=Matrix(K*u)  SaturateOnIntegerOverflow=on  OutDataTypeStr=Inherit: Same as input  ParamDataTypeStr=Inherit: Same as input
  3x3 Cross Product : Subsystem  AncestorBlock=aerolibtransform/3x3 Cross Product  mask(CrossProduct){}
      mask help: Calculate the cross product of two 3-by-1 vectors.
      mask Help: web(asbhelp('3x3crossproduct'));
      mask Display: disp('Cross Product \n C = AxB')
  Clock : Clock
  DWN : Gain  Gain=DWN  Multiplication=Matrix(K*u)  SaturateOnIntegerOverflow=on  OutDataTypeStr=Inherit: Same as input  ParamDataTypeStr=Inherit: Same as input
  DWN1 : Gain  Gain=DWN  Multiplication=Matrix(K*u)  SaturateOnIntegerOverflow=on  OutDataTypeStr=Inherit: Same as input  ParamDataTypeStr=Inherit: Same as input
  DWN2 : Gain  Gain=DWN  Multiplication=Matrix(K*u)  SaturateOnIntegerOverflow=on  OutDataTypeStr=Inherit: Same as input  ParamDataTypeStr=Inherit: Same as input
  IW : Gain  Gain=IW  SaturateOnIntegerOverflow=on  OutDataTypeStr=Inherit: Same as input  ParamDataTypeStr=Inherit: Same as input
  JW : Gain  Gain=JW  SaturateOnIntegerOverflow=on  OutDataTypeStr=Inherit: Same as input  ParamDataTypeStr=Inherit: Same as input
  Mux : Mux
  Product : Product  SaturateOnIntegerOverflow=on  InputSameDT=on  OutDataTypeStr=Inherit: Same as first input
  Product1 : Product  SaturateOnIntegerOverflow=on  InputSameDT=on  OutDataTypeStr=Inherit: Same as first input
  Product2 : Product  SaturateOnIntegerOverflow=on  InputSameDT=on  OutDataTypeStr=Inherit: Same as first input
  Scope{1..6} (6 alike) : Scope
  Sum : Sum  Inputs=|+-  SaturateOnIntegerOverflow=on
  Sum1 : Sum  Inputs=|+|+|+|  SaturateOnIntegerOverflow=on  InputSameDT=on  OutDataTypeStr=Inherit: Same as first input
  Trigonometric Function : Trigonometry  Operator=cos
  Unit delay : UnitDelay  InitialCondition=HWw0  SampleTime=0.05
  TW : Outport
  wires:
  JW/1 -> DWN1/1, Sum/2, Scope2/1, Unit delay/1
  Wb/1 -> 3x3 Cross Product/2(B)
  DWN1/1 -> 3x3 Cross Product/1(A)
  Clock/1 -> Mux/1, Mux/3, Mux/4, Mux/2
  Mux/1 -> Product/1
  Ew/1 -> JW/1, Product1/1, Product1/2, Product/2
  Product1/1 -> IW/1
  Product/1 -> Trigonometric Function/1
  IW/1 -> Product2/1
  Trigonometric Function/1 -> Product2/2
  Product2/1 -> DWN2/1
  DWN2/1 -> Sum1/3, Scope4/1
  Sum1/1 -> Scope6/1, TW/1
  DWN/1 -> Scope3/1, Sum1/1
  3x3 Cross Product/1(C) -> Sum1/2, Scope5/1
  Unit delay/1 -> Sum/1
  Sum/1 -> Scope1/1, 1/T/1
  1/T/1 -> DWN/1

== system fangzhen20200803/Dynamics System动力系统/Attitude姿态/反作用飞轮/wheelmid ==
  note: 角速度
  note: 角动量
  note: 力矩
  Uwheel : Inport
  CWw : Gain  Gain=CWw  SaturateOnIntegerOverflow=on  OutDataTypeStr=Inherit: Same as input  ParamDataTypeStr=Inherit: Same as input
  Constant2 : Constant  Value=[0 0 0 0]
  Data Type Conversion1 : DataTypeConversion  OutDataTypeStr=double  SaturateOnIntegerOverflow=on  RndMeth=Zero
  Data Type Conversion2 : DataTypeConversion  OutDataTypeStr=double  SaturateOnIntegerOverflow=on  RndMeth=Zero
  Discrete-Time Integrator : DiscreteIntegrator  InitialCondition=HWw0  SampleTime=0.05  LimitOutput=on  UpperSaturationLimit=Hwmax  LowerSaturationLimit=-Hwmax  ICPrevOutput=DiscIntNeverNeededParam  ICPrevScaledInput=DiscIntNeverNeededParam
  R1 : Scope
  R3 : Scope
  Relational Operator : RelationalOperator  Operator=>  RndMeth=Nearest  InputSameDT=on
  Relational Operator1 : RelationalOperator  Operator=<  RndMeth=Nearest  InputSameDT=on
  Saturation : Saturate  UpperLimit=Tcmax  LowerLimit=-Tcmax
  Sum : Sum  SaturateOnIntegerOverflow=on  InputSameDT=on  OutDataTypeStr=Inherit: Same as first input
  Sum1 : Sum  Inputs=|+|-|-|  SaturateOnIntegerOverflow=on  InputSameDT=on  OutDataTypeStr=Inherit: Same as first input
  Sum2 : Sum  Inputs=+-  SaturateOnIntegerOverflow=on  InputSameDT=on  OutDataTypeStr=Inherit: Same as first input
  TWi : RandomNumber  Mean=[0 0 0 0]  Variance=[0 0 0 0]  Seed=[0 0 0 0]  SampleTime=0
  Tf0 : Gain  Gain=TWf0  SaturateOnIntegerOverflow=on  OutDataTypeStr=Inherit: Same as input  ParamDataTypeStr=Inherit: Same as input
  invJW : Gain  Gain=invJW  SaturateOnIntegerOverflow=on  OutDataTypeStr=Inherit: Same as input  ParamDataTypeStr=Inherit: Same as input
  Ww : Outport
  wires:
  TWi/1 -> Sum1/1
  Sum1/1 -> Sum/2, R3/1
  invJW/1 -> R1/1, Ww/1, Relational Operator/1, CWw/1, Relational Operator1/1
  Relational Operator/1 -> Data Type Conversion1/1
  Relational Operator1/1 -> Data Type Conversion2/1
  Sum2/1 -> Tf0/1
  Tf0/1 -> Sum1/3
  CWw/1 -> Sum1/2
  Uwheel/1 -> Saturation/1
  Sum/1 -> Discrete-Time Integrator/1
  Discrete-Time Integrator/1 -> invJW/1
  Saturation/1 -> Sum/1
  Constant2/1 -> Relational Operator/2, Relational Operator1/2
  Data Type Conversion1/1 -> Sum2/1
  Data Type Conversion2/1 -> Sum2/2

== system fangzhen20200803/Dynamics System动力系统/Attitude姿态/姿态动力学模型/3x3 Cross Product ==
  A : Inport
  B : Inport  Port=2
  Product : Product  SaturateOnIntegerOverflow=on  InputSameDT=on  OutDataTypeStr=Inherit: Same as first input
  Product1 : Product  SaturateOnIntegerOverflow=on  InputSameDT=on  OutDataTypeStr=Inherit: Same as first input
  Selector : Selector  InputPortWidth=3  IndexOptions=Index vector (dialog)  Indices=[2 3 1]  OutputSizes=1
  Selector1 : Selector  InputPortWidth=3  IndexOptions=Index vector (dialog)  Indices=[3 1 2]  OutputSizes=1
  Selector2 : Selector  InputPortWidth=3  IndexOptions=Index vector (dialog)  Indices=[2 3 1]  OutputSizes=1
  Selector3 : Selector  InputPortWidth=3  IndexOptions=Index vector (dialog)  Indices=[3 1 2]  OutputSizes=1
  Sum : Sum  Inputs=+|-  SaturateOnIntegerOverflow=on  InputSameDT=on  OutDataTypeStr=Inherit: Same as first input
  C : Outport  InitialOutput=0
  wires:
  Sum/1 -> C/1
  B/1 -> Selector1/1, Selector2/1
  Selector/1 -> Product/1
  A/1 -> Selector/1, Selector3/1
  Product/1 -> Sum/1
  Selector1/1 -> Product/2
  Product1/1 -> Sum/2
  Selector2/1 -> Product1/2
  Selector3/1 -> Product1/1

== system fangzhen20200803/Dynamics System动力系统/Orbit轨道/轨道动力学模型/哥式惯性加速度 ==
  v : Inport
  Matrix Gain : Gain  Gain=-B  Multiplication=Matrix(K*u)  SaturateOnIntegerOverflow=on  OutDataTypeStr=Inherit: Same as input  ParamDataTypeStr=Inherit: Same as input
  -ak : Outport
  wires:
  v/1 -> Matrix Gain/1
  Matrix Gain/1 -> -ak/1

== system fangzhen20200803/Dynamics System动力系统/Orbit轨道/轨道动力学模型/小行星引力加速度 ==
  r : Inport
  Matrix Gain : Gain  Gain=Tl'  Multiplication=Matrix(K*u)  SaturateOnIntegerOverflow=on  OutDataTypeStr=Inherit: Same as input  ParamDataTypeStr=Inherit: Same as input
  Matrix Gain1 : Gain  Gain=Gl  Multiplication=Matrix(K*u)  SaturateOnIntegerOverflow=on  OutDataTypeStr=Inherit: Same as input  ParamDataTypeStr=Inherit: Same as input
  Matrix Gain2 : Gain  Gain=Gl'  Multiplication=Matrix(K*u)  SaturateOnIntegerOverflow=on  OutDataTypeStr=Inherit: Same as input  ParamDataTypeStr=Inherit: Same as input
  Sum : Sum  SaturateOnIntegerOverflow=on
  "[0;0;R0]" : Constant  Value=R0
  小行星引力 : Subsystem
      mask Display: disp('小行星引力')
  U : Outport
  wires:
  r/1 -> Matrix Gain/1
  Matrix Gain/1 -> Sum/1
  "[0;0;R0]"/1 -> Sum/2
  Sum/1 -> Matrix Gain1/1
  Matrix Gain1/1 -> 小行星引力/1(r')
  小行星引力/1(U) -> Matrix Gain2/1
  Matrix Gain2/1 -> U/1

== system fangzhen20200803/Dynamics System动力系统/Orbit轨道/轨道动力学模型/离心惯性加速度 ==
  r : Inport
  Matrix Gain : Gain  Gain=-A  Multiplication=Matrix(K*u)  SaturateOnIntegerOverflow=on  OutDataTypeStr=Inherit: Same as input  ParamDataTypeStr=Inherit: Same as input
  R0 : Constant  Value=R0
  Sum : Sum  SaturateOnIntegerOverflow=on
  -ae : Outport
  wires:
  r/1 -> Sum/1
  R0/1 -> Sum/2
  Sum/1 -> Matrix Gain/1
  Matrix Gain/1 -> -ae/1

== system fangzhen20200803/GNC System/喷嘴控制器1/detR+/Switch ==
  detV : Inport
  Constant : Constant  Value=-d+b
  Constant1 : Constant  Value=-d
  Gain : Gain  Gain=-1/2/a0  SaturateOnIntegerOverflow=on  OutDataTypeStr=Inherit: Same as input  ParamDataTypeStr=Inherit: Same as input
  Gain1 : Gain  Gain=1/2/a  SaturateOnIntegerOverflow=on  OutDataTypeStr=Inherit: Same as input  ParamDataTypeStr=Inherit: Same as input
  Math Function : Math  Operator=magnitude^2  SaturateOnIntegerOverflow=on
  Sum : Sum  SaturateOnIntegerOverflow=on
  Sum1 : Sum  SaturateOnIntegerOverflow=on
  Out1 : Outport
  Out2 : Outport  Port=2
  wires:
  Math Function/1 -> Gain/1, Gain1/1
  Gain/1 -> Sum/2
  Constant/1 -> Sum/1
  Gain1/1 -> Sum1/1
  Constant1/1 -> Sum1/2
  detV/1 -> Math Function/1
  Sum/1 -> Out1/1
  Sum1/1 -> Out2/1

== system fangzhen20200803/GNC System/喷嘴控制器1/detR-/Switch ==
  detV : Inport
  Constant : Constant  Value=d
  Constant1 : Constant  Value=d-b
  Gain : Gain  Gain=-1/2/a  SaturateOnIntegerOverflow=on  OutDataTypeStr=Inherit: Same as input  ParamDataTypeStr=Inherit: Same as input
  Gain1 : Gain  Gain=1/2/a0  SaturateOnIntegerOverflow=on  OutDataTypeStr=Inherit: Same as input  ParamDataTypeStr=Inherit: Same as input
  Math Function : Math  Operator=magnitude^2  SaturateOnIntegerOverflow=on
  Sum : Sum  SaturateOnIntegerOverflow=on
  Sum1 : Sum  SaturateOnIntegerOverflow=on
  Out1 : Outport
  Out2 : Outport  Port=2
  wires:
  detV/1 -> Math Function/1
  Math Function/1 -> Gain/1, Gain1/1
  Gain/1 -> Sum/2
  Constant/1 -> Sum/1
  Sum/1 -> Out1/1
  Gain1/1 -> Sum1/1
  Constant1/1 -> Sum1/2
  Sum1/1 -> Out2/1

== system fangzhen20200803/GNC System/导航与滤波/Calculate/P1 ==
  In1 : Inport
  Constant : Constant  Value=f
  Fcn : Fcn  Expr=u[3]/(u[1]^2+u[2]^2+f^2)^0.5
  Fcn1 : Fcn  Expr=u[1]
  Fcn2 : Fcn  Expr=u[2]
  Mux : Mux  Inputs=3
  Product : Product  SaturateOnIntegerOverflow=on  OutDataTypeStr=Inherit: Same as first input
  Out1 : Outport
  wires:
  In1/1 -> Fcn1/1, Fcn/1, Fcn2/1
  Fcn/1 -> Product/2
  Product/1 -> Out1/1
  Fcn1/1 -> Mux/1
  Fcn2/1 -> Mux/2
  Constant/1 -> Mux/3
  Mux/1 -> Product/1

== system fangzhen20200803/GNC System/导航与滤波/Calculate/P2 ==
  In1 : Inport
  Constant : Constant  Value=f
  Fcn : Fcn  Expr=u[3]/(u[1]^2+u[2]^2+f^2)^0.5
  Fcn1 : Fcn  Expr=u[1]
  Fcn2 : Fcn  Expr=u[2]
  Mux : Mux  Inputs=3
  Product : Product  SaturateOnIntegerOverflow=on  OutDataTypeStr=Inherit: Same as first input
  Out1 : Outport
  wires:
  Mux/1 -> Product/1
  Constant/1 -> Mux/3
  Fcn2/1 -> Mux/2
  Fcn1/1 -> Mux/1
  Product/1 -> Out1/1
  Fcn/1 -> Product/2
  In1/1 -> Fcn2/1, Fcn/1, Fcn1/1

== system fangzhen20200803/GNC System/导航与滤波/Calculate/P3 ==
  In1 : Inport
  Constant : Constant  Value=f
  Fcn : Fcn  Expr=u[3]/(u[1]^2+u[2]^2+f^2)^0.5
  Fcn1 : Fcn  Expr=u[1]
  Fcn2 : Fcn  Expr=u[2]
  Mux : Mux  Inputs=3
  Product : Product  SaturateOnIntegerOverflow=on  OutDataTypeStr=Inherit: Same as first input
  Out1 : Outport
  wires:
  In1/1 -> Fcn1/1, Fcn/1, Fcn2/1
  Fcn/1 -> Product/2
  Product/1 -> Out1/1
  Fcn1/1 -> Mux/1
  Fcn2/1 -> Mux/2
  Constant/1 -> Mux/3
  Mux/1 -> Product/1
